simulink model "estnieuw"  (R2026a)
settings: Solver=VariableStepAuto  StopTime=31535100
values from neighbouring files (symbols this model uses):
  eta_turbine = 0.4    [run_estnieuw_outputs.m]
  R_line = 30    [run_estnieuw_outputs.m]
  V_line = 220e3    (= 220000)    [run_estnieuw_outputs.m]
libraries: fl_lib x5, nesl_utility x4, simulink x1
settings Model: Creator=user  LastModifiedBy=flin
settings SimscapeCC: SimscapeNominalValues="[{\"value\":\"1\",\"unit\":\"A\"},{\"value\":\"1\",\"unit\":\"bar\"},{\"value\":\"1\",\"unit\":\"cm^2\"},{\"value\":\"1\",\"unit\":\"cm^3/s\"},{\"value\":\"1\",\"unit\":\"kJ/kg\"},{\"value\":\"1\",\"unit\":\"kW\"},{\"value\":\"1\",\"unit\":\"l\"},{\"value\":\"1\",\"unit\":\"N\"},{\"value\":\"1\",\"unit\":\"N*m\"},{\"value\":\"1\",\"unit\":\"V\"}]"  SimscapeLogType=none  SimscapeLogDataHistory=5000.0

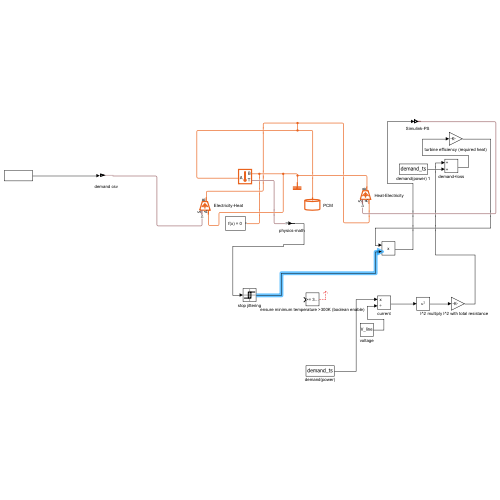
[thumbnail: Simulink's stored preview of the top-level diagram]
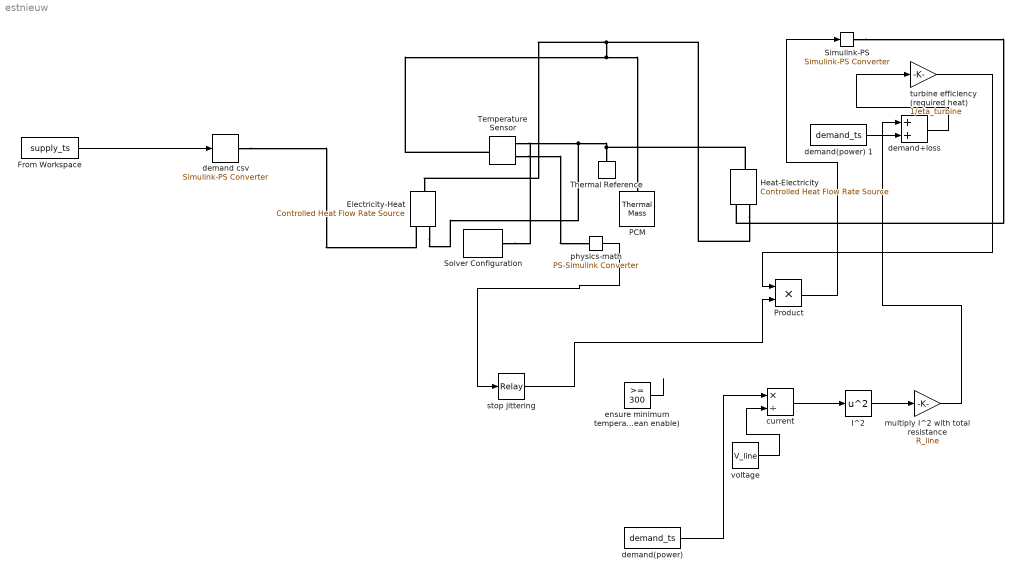
== system estnieuw ==
  Electricity-Heat : fl_lib/Thermal/Thermal Sources/Controlled Heat Flow Rate Source
  From Workspace : FromWorkspace  VariableName=supply_ts
  Heat-Electricity : fl_lib/Thermal/Thermal Sources/Controlled Heat Flow Rate Source
  I^2 : Math  Operator=square
  PCM : fl_lib/Thermal/Thermal Elements/Thermal Mass  mass_type=foundation.enum.constant_variable.constant  mass=2.8e6 kg  sp_heat=1600 J/(K*kg)  mass_min=1e-6 kg  num_ports=foundation.enum.numPorts2.one  m_specify=off  m_priority=High  m=1 kg  m_nominal_specify=off  m_nominal_value=1  m_nominal_unit=kg  T_specify=on  T_priority=High  T=600 K  T_nominal_specify=off  T_nominal_value=773.15  T_nominal_unit=K  Q_specify=off  Q_priority=None  Q=0 W  Q_nominal_specify=off  Q_nominal_value=1  Q_nominal_unit=W
  Product : Product
  "Simulink-PS " : nesl_utility/Simulink-PS Converter  PhysicalDomain=network_engine_domain  SubClassName=ps_input  LeftPortType=input  RightPortType=output  PseudoPeriodic=off  Frequencies=[]  NoiseDistribution=none  NoiseParameters=[]  Unit=W  AffineConversion=off  FilteringAndDerivatives=provide  SimscapeFilterOrder=1  InputFilterTimeConstant=0.001  UdotUserProvided=0
  Solver Configuration : nesl_utility/Solver Configuration  PhysicalDomain=network_engine_domain  SubClassName=solver  LeftPortType=input  RightPortType=generic  Tones=[]  Harmonics=[]  SimulateNoise=off  Profile=off  UseLocalSampling=off  EnableSwitchedLinearOptims=on  FrequencyDomain=off  UseCCode=off  RelTol=0.001  AbsTol=0.001  MinStep=1e-09  ToWorkspace=off  RevertToSquareIcSolve=off  NumHomotopyIterations=100  PhasorMode=off  PhasorModeNumHarmonics=1  ConsistencySolver=NEWTON_XTOL_AFTER_FTOL  CanonicalOrdering=UNORDERED  OptimizeIntermediates=UNOPTIMIZED  IndexReductionMethod=DerivativeReplacement  DoDC=off  ResidualTolerance=1e-09  ConsistencyTolSource=GLOBAL  ConsistencyAbsTol=0.001  ConsistencyRelTol=0.001  ConsistencyTolFactor=0.001  UseLocalSolver=off  LocalSolverChoice=NE_BACKWARD_EULER_ADVANCER  ResolveIndetEquations=on  FunctionEvalNumThread=1  LocalSolverSampleTime=0.001  DoFixedCost=off  MaxNonlinIter=3  MaxModeIter=2  ComputeImpulses=off  ImpulseIterations=2  LinearAlgebra=auto  LinearAlgebraNumThread=0  EquationFormulation=NE_TIME_EF  DelaysMemoryBudget=1024  AutomaticFiltering=on  FilteringTimeConstant=0.001  PartitionStorageMethod=AS_NEEDED  PartitionMemoryBudget=1024  PartitionMethod=ROBUST  MultibodyUseLocalSolver=off  MultibodyLocalSolverChoice=ODE1  MultibodyLocalSolverSampleTime=0.001
  Temperature Sensor : fl_lib/Thermal/Thermal Sensors/Temperature Sensor  temperature_measure=foundation.enum.MeasurementReference.difference
  Thermal Reference : fl_lib/Thermal/Thermal Elements/Thermal Reference
  current : Product  Inputs=*/
  demand csv : nesl_utility/Simulink-PS Converter  PhysicalDomain=network_engine_domain  SubClassName=ps_input  LeftPortType=input  RightPortType=output  PseudoPeriodic=off  Frequencies=[]  NoiseDistribution=none  NoiseParameters=[]  Unit=W  AffineConversion=off  FilteringAndDerivatives=provide  SimscapeFilterOrder=1  InputFilterTimeConstant=0.001  UdotUserProvided=0
  demand(power) : FromWorkspace  VariableName=demand_ts
  demand(power) 1 : FromWorkspace  VariableName=demand_ts
  demand+loss : Sum
  ensure minimum temperature >300K (boolean enable) : simulink/Logic and Bit Operations/Compare To Constant  relop=>=  const=300  OutDataTypeStr=boolean
  multiply I^2 with total resistance : Gain  Gain=R_line
  physics-math : nesl_utility/PS-Simulink Converter  PhysicalDomain=network_engine_domain  SubClassName=ps_output  LeftPortType=input  RightPortType=output  PseudoPeriodic=off  Frequencies=[]  VectorFormat=inherit  Unit=K  AffineConversion=off
  stop jittering : Relay  OnSwitchValue=310  OffSwitchValue=300
  turbine efficiency (required heat) : Gain  Gain=1/eta_turbine
  voltage : Constant  Value=V_line
  wires:
  demand(power)/1 -> current/1
  current/1 -> I^2/1
  I^2/1 -> multiply I^2 with total resistance/1
  voltage/1 -> current/2
  multiply I^2 with total resistance/1 -> demand+loss/1
  demand(power) 1/1 -> demand+loss/2
  demand+loss/1 -> turbine efficiency (required heat)/1
  turbine efficiency (required heat)/1 -> Product/1
  From Workspace/1 -> demand csv/1
  physics-math/1 -> stop jittering/1
  ensure minimum temperature >300K (boolean enable)/1 -> ?
  Product/1 -> "Simulink-PS "/1
  stop jittering/1 -> Product/2
  connections:
  Solver Configuration/RConn1 -- Temperature Sensor/RConn1 -- Electricity-Heat/RConn2 -- Thermal Reference/LConn1 -- Heat-Electricity/LConn1
  Heat-Electricity/RConn2 -- Electricity-Heat/LConn1 -- Temperature Sensor/LConn1 -- PCM/LConn1
  demand csv/RConn1 -- Electricity-Heat/RConn1
  Temperature Sensor/RConn2 -- physics-math/LConn1
  "Simulink-PS "/RConn1 -- Heat-Electricity/RConn1
